simulink model "simpleFeedback"  (R2022b)
settings: Solver=VariableStepAuto  StartTime=0.0  StopTime=10.0  RelTol=1e-3
values from neighbouring files (symbols this model uses):
  K = K_test(i)    [simpleFeedback.m]
settings Model: Creator=sooru  LastModifiedBy=sooru

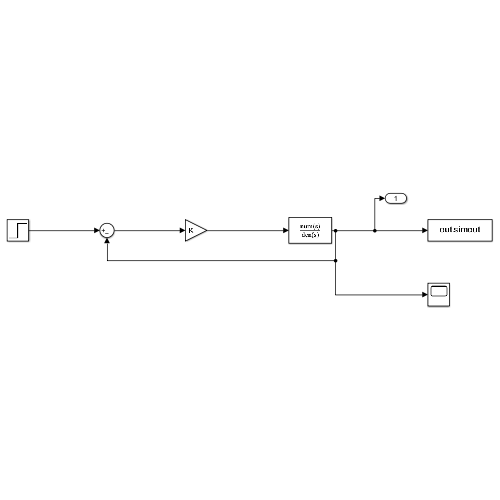
[thumbnail: Simulink's stored preview of the top-level diagram]
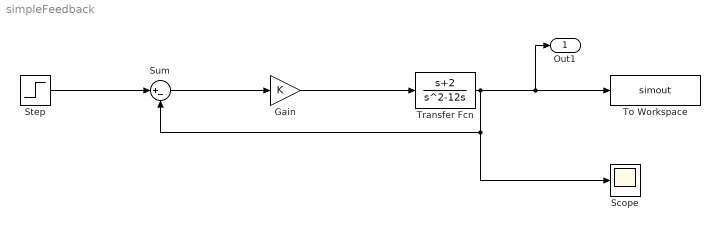
== system simpleFeedback ==
  Gain : Gain  Gain=K
  Scope : Scope
  Step : Step  Time=0  SampleTime=0
  Sum : Sum  Inputs=|+-
  To Workspace : ToWorkspace  VariableName=simout  SaveFormat=Timeseries  SampleTime=-1
  Transfer Fcn : TransferFcn  Numerator=[1 2]  Denominator=[1 -12 0]
  Out1 : Outport
  wires:
  Step/1 -> Sum/1
  Sum/1 -> Gain/1
  Gain/1 -> Transfer Fcn/1
  Transfer Fcn/1 -> Scope/1, Sum/2, Out1/1, To Workspace/1
